simulink model "Plantnl"  (Simulink 7.9)
settings: Solver=ode45  SolverMode=SingleTasking  StartTime=0.0  StopTime=100  RelTol=1e-3  AbsTol=1e-6
undefined symbols (not defined in the file or in its folder): Conduction, InputFlux, M_inv, Radiation, ScaleTemp
settings Model: Creator=abbas  LastModifiedBy=abbas
settings DataIOCC: LimitDataPoints=off
settings OptimizationCC: BlockReduction=off  BooleanDataType=off  InlineInvariantSignals=on  InitFltsAndDblsToZero=on
settings DebuggingCC: SaveWithParameterizedLinksMsg=none  SignalResolutionControl=TryResolveAllWithWarning  SolverPrmCheckMsg=none  MultiTaskDSMMsg=warning  MultiTaskCondExecSysMsg=none  FcnCallInpInsideContextMsg=Use local settings  StrictBusMsg=None
settings HardwareCC: TargetUnknown=on
settings RTWCC: IncludeERTFirstTime=on
settings GRTTargetCC: TargetFcnLib=ansi_tfl_tmw.mat  ModelReferenceCompliant=off  CompOptLevelCompliant=off  CombineOutputUpdateFcns=off  MatFileLogging=off  GRTInterface=on

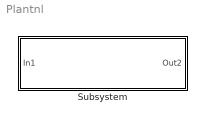
== system Plantnl ==
  Subsystem : Subsystem

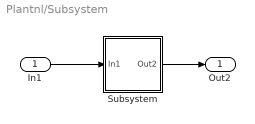
== system Plantnl/Subsystem ==
  In1 : Inport
  Subsystem : Subsystem
  Out2 : Outport
  wires:
  In1/1 -> Subsystem/1(In1)
  Subsystem/1(Out2) -> Out2/1

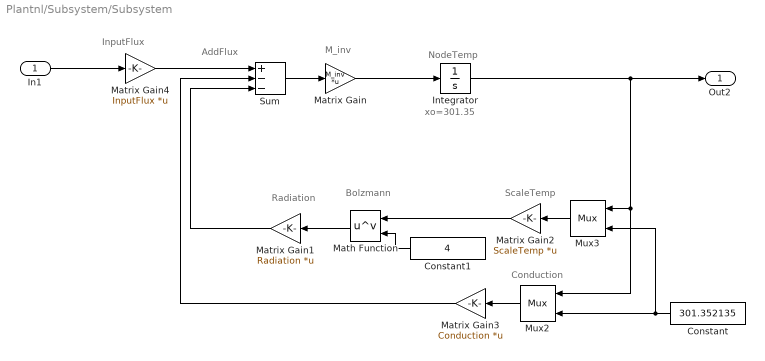
== system Plantnl/Subsystem/Subsystem ==
  note: InputFlux
  note: AddFlux
  note: M_inv
  note: NodeTemp
  note: xo=301.35
  note: Radiation
  note: ScaleTemp
  note: Conduction
  note: Bolzmann
  In1 : Inport
  Constant : Constant  Value=301.352135
  Constant1 : Constant  Value=4
  Integrator : Integrator  InitialCondition=301.3521350999999
  Math Function : Math  Operator=pow  SaturateOnIntegerOverflow=on
  Matrix Gain : Gain  Gain=M_inv  Multiplication=Matrix(K*u)  SaturateOnIntegerOverflow=on  OutDataTypeStr=Inherit: Same as input  ParamDataTypeStr=Inherit: Same as input
  Matrix Gain1 : Gain  Gain=Radiation  Multiplication=Matrix(K*u)  SaturateOnIntegerOverflow=on  OutDataTypeStr=Inherit: Same as input  ParamDataTypeStr=Inherit: Same as input
  Matrix Gain2 : Gain  Gain=ScaleTemp  Multiplication=Matrix(K*u)  SaturateOnIntegerOverflow=on  OutDataTypeStr=Inherit: Same as input  ParamDataTypeStr=Inherit: Same as input
  Matrix Gain3 : Gain  Gain=Conduction  Multiplication=Matrix(K*u)  SaturateOnIntegerOverflow=on  OutDataTypeStr=Inherit: Same as input  ParamDataTypeStr=Inherit: Same as input
  Matrix Gain4 : Gain  Gain=InputFlux  Multiplication=Matrix(K*u)  SaturateOnIntegerOverflow=on  OutDataTypeStr=Inherit: Same as input  ParamDataTypeStr=Inherit: Same as input
  Mux2 : Mux  Inputs=2
  Mux3 : Mux  Inputs=2
  Sum : Sum  Inputs=+--  SaturateOnIntegerOverflow=on  InputSameDT=on  OutDataTypeStr=Inherit: Same as first input
  Out2 : Outport
  wires:
  Matrix Gain4/1 -> Sum/1
  Sum/1 -> Matrix Gain/1
  Matrix Gain/1 -> Integrator/1
  Integrator/1 -> Mux2/1, Mux3/1, Out2/1
  Mux3/1 -> Matrix Gain2/1
  Mux2/1 -> Matrix Gain3/1
  Matrix Gain3/1 -> Sum/2
  Constant/1 -> Mux2/2, Mux3/2
  Matrix Gain1/1 -> Sum/3
  Math Function/1 -> Matrix Gain1/1
  Matrix Gain2/1 -> Math Function/1
  Constant1/1 -> Math Function/2
  In1/1 -> Matrix Gain4/1
